simulink model "Control_model_10DOF_fin"  (R2016b)
settings: Solver=FixedStepAuto  StartTime=0.0  StopTime=10  FixedStep=0.0001  RelTol=1e-3
InitFcn:
  | Initialisation_ctr_10DOF_fin
values from neighbouring files (symbols this model uses):
  COM_Parameters = [-lpelvis/2;r2;0]    [Initialisation_ctr_10DOF_fin.m]
  DH_Parameters = [hfoot 0 ... (first row only)    [Initialisation_ctr_10DOF_fin.m]
  dTrunk = trunklbd(3)    [Initialisation_ctr_10DOF_fin.m]
  dxFootSM = dxFoot    [Initialisation_ctr_10DOF_fin.m]
  dxTrunk = 0.1    [Initialisation_ctr_10DOF_fin.m]
  Foot_Parameters = [0;-(lFoot/2-lHeel);0]    [Initialisation_ctr_10DOF_fin.m]
  HAA2HEE = [0; 0; 0.001]    [Initialisation_ctr_10DOF_fin.m]
  HEE2HFE = 0.5*[0.2; 0; 0]    [Initialisation_ctr_10DOF_fin.m]
  height_vrp = CoM_position(1)    [Initialisation_ctr_10DOF_fin.m]
  hTrunk = trunklbd(1)    [Initialisation_ctr_10DOF_fin.m]
  initial_CoM_position = R*CoM_position    [Initialisation_ctr_10DOF_fin.m]
  initial_CoM_velocity = [0;0;0]    [Initialisation_ctr_10DOF_fin.m]
  initial_left_foot = [0;0;-stance_width/2]    [Initialisation_ctr_10DOF_fin.m]
  initial_right_foot = [0;0;stance_width/2]    [Initialisation_ctr_10DOF_fin.m]
  initial_RorL = 0    [Initialisation_ctr_10DOF_fin.m]
  jointsinitial = [9;-15;6;0;0;6;-15;9]/180*pi    [Initialisation_ctr_10DOF_fin.m]
  K_DCM = 4.3*[1 0 0 ... (first row only)    [Initialisation_ctr_10DOF_fin.m]
  kD_left = mbody*[0.95 0 0 0 ... (first row only)    [Initialisation_ctr_10DOF_fin.m]
  kD_right = mbody*[0.12 0 0 0 ... (first row only)    [Initialisation_ctr_10DOF_fin.m]
  kI_left = mbody*[35 0 0 0 ... (first row only)    [Initialisation_ctr_10DOF_fin.m]
  kI_right = mbody*[38.2 0 0 0 ... (first row only)    [Initialisation_ctr_10DOF_fin.m]
  kP_left = mbody*[75 0 0 0 ... (first row only)    [Initialisation_ctr_10DOF_fin.m]
  kP_right = mbody*[5.6 0 0 0 ... (first row only)    [Initialisation_ctr_10DOF_fin.m]
  Lenght = [lShank;lThigh]    [Initialisation_ctr_10DOF_fin.m]
  lFootSM = lFoot    [Initialisation_ctr_10DOF_fin.m]
  lpelvis = wPelvis    [Initialisation_ctr_10DOF_fin.m]
  mass = mbody    (= 60)    [Initialisation_ctr_10DOF_fin.m]
  Masses = [mThigh; mShank; mTrunk]    [Initialisation_ctr_10DOF_fin.m]
  nb_step = 4    [Initialisation_ctr_10DOF_fin.m]
  nb_step_pattern = 20    [Initialisation_ctr_10DOF_fin.m]
  Pelvis_Parameters = [-lpelvis/2;hTrunk/2;0]    [Initialisation_ctr_10DOF_fin.m]
  stance_width = lpelvis    [Initialisation_ctr_10DOF_fin.m]
  stride_lenght = 0.50    (= 0.5)    [Initialisation_ctr_10DOF_fin.m]
  T_DS = time_DS    (= 0.4)    [Initialisation_ctr_10DOF_fin.m]
  T_IT = time_DS    (= 0.4)    [Initialisation_ctr_10DOF_fin.m]
  T_SS = time_swing    (= 1.6)    [Initialisation_ctr_10DOF_fin.m]
  time_DS = (time_stance-time_swing)/2    (= 0.4)    [Initialisation_ctr_10DOF_fin.m]
  time_stance = 60/100*time_stride    (= 2.4)    [Initialisation_ctr_10DOF_fin.m]
  time_step = time_stride/2    (= 2)    [Initialisation_ctr_10DOF_fin.m]
  time_swing = 40/100*time_stride    (= 1.6)    [Initialisation_ctr_10DOF_fin.m]
  validity_angle = [-20*pi/180 20*pi/180 ... (first row only)    [Initialisation_ctr_10DOF_fin.m]
  wTrunk = trunklbd(2)    [Initialisation_ctr_10DOF_fin.m]
  x4CoM = CoM_position(1)-XR4(1)    [Initialisation_ctr_10DOF_fin.m]
undefined symbols (not defined in the file or in its folder): dsegment, hFoot, l, lFoot, omega0_x, omega0_z, rho, wPelvis, X, Xp_x, Xp_z, Y, Z
undefined symbols (not defined in the file): k_grf, lShankSM, lThighSM, mShank, mThigh
libraries: nesl_utility x247, sm_lib x215, dspindex x12, FootPlacementLibrary x8, dspsigops x4, dspswit3 x1
(part 14 of 18)

== matlab function Control_model_10DOF_fin/10DoF Walker SimMechanics Model/Knee FE/MATLAB Function ==
  data: joint input; velocity input; desired_torque input; torque output; validity_angle parameter
function torque = fcn(joint,velocity,desired_torque,validity_angle)

kp=900;
kv=0.008;

min=validity_angle(2,1);
max=validity_angle(2,2);

if joint<=min
    torque=kp*(min-joint)-kv*velocity;
    if torque<=0
        torque=desired_torque;
    end
elseif joint>=max
    torque=kp*(max-joint)-kv*velocity;
    if torque>=0
        torque=desired_torque;
    end
else
    torque=desired_torque;
end

== matlab function Control_model_10DOF_fin/10DoF Walker SimMechanics Model/Knee FE1/MATLAB Function ==
  data: joint input; velocity input; desired_torque input; torque output; validity_angle parameter
function torque = fcn(joint,velocity,desired_torque,validity_angle)

kp=900;
kv=0.008;

min=validity_angle(7,1);
max=validity_angle(7,2);

if joint<=min
    torque=kp*(min-joint)-kv*velocity;
    if torque<=0
        torque=desired_torque;
    end
elseif joint>=max
    torque=kp*(max-joint)-kv*velocity;
    if torque>=0
        torque=desired_torque;
    end
else
    torque=desired_torque;
end

== matlab function Control_model_10DOF_fin/Control/Double_Support/Left stance phase1/Subsystem/MATLAB Function1 ==
  data: r_vrp_W input size=3; TWR input; TWL input; lFoot parameter; dsegment parameter; new_vrp_W output; alpha output
function [new_vrp_W,alpha]  = support_polygon(r_vrp_W,TWR,TWL,lFoot,dsegment)


RWL=TWL(1:3,1:3);
Left_foot_position=TWL(1:3,4);
Right_foot_position=TWR(1:3,4);

p=85/100;

R1W=Right_foot_position+RWL*[0;-lFoot/2;-dsegment/2]*p;
R2W=Right_foot_position+RWL*[0;-lFoot/2;dsegment/2]*p;
R3W=Right_foot_position+RWL*[0;lFoot/2;dsegment/2]*p;
R4W=Right_foot_position+RWL*[0;lFoot/2;-dsegment/2]*p;

L1W=Left_foot_position+RWL*[0;-lFoot/2;-dsegment/2]*p;
L2W=Left_foot_position+RWL*[0;-lFoot/2;dsegment/2]*p;
L3W=Left_foot_position+RWL*[0;lFoot/2;dsegment/2]*p;
L4W=Left_foot_position+RWL*[0;lFoot/2;-dsegment/2]*p;

dR=norm(r_vrp_W-Right_foot_position);
dL=norm(r_vrp_W-Left_foot_position);

alpha=dR/(dR+dL);
% if Right_foot_position(2)>0
%     alpha=1;
% end

% Projection on the ground
R1W(2)=0;
R2W(2)=0;
R3W(2)=0;
R4W(2)=0;

L1W(2)=0;
L2W(2)=0;
L3W(2)=0;
L4W(2)=0;

% New frame

x=1/norm(L1W-L4W)*(L1W-L4W);
y=[0;1;0];
z=1/norm(L2W-L1W)*(L2W-L1W);

R=[x,y,z];

% Points on the Left foot origin and new frame


L1=R.'*(L1W-Left_foot_position);
L2=R.'*(L2W-Left_foot_position);
L3=R.'*(L3W-Left_foot_position);
L4=R.'*(L4W-Left_foot_position);

% VRP and DCM on the left foot origin and new frame

r_vrp=R.'*(r_vrp_W-Left_foot_position);


outside=1;

if r_vrp(1)<L1(1) && r_vrp(3)>L1(3) && r_vrp(1)>L3(1) && r_vrp(3)<L3(3)
    outside=0;
    alpha=0;
end

cas=0;

new_vrp=r_vrp;

if outside==1
    if r_vrp(1)>=L1(1) && r_vrp(3)<=L1(3)
        new_vrp(1)=L1(1);
        new_vrp(3)=L1(3);
    elseif r_vrp(1)>=L2(1) && r_vrp(3)>=L2(3)
        new_vrp(1)=L2(1);
        new_vrp(3)=L2(3);
    elseif r_vrp(1)>=L1(1)
        new_vrp(1)=L1(1);
    elseif r_vrp(1)<=L3(1) && r_vrp(3)>=L3(3)
        new_vrp(1)=L3(1);
        new_vrp(3)=L3(3);
    elseif r_vrp(3)>=L3(3)
        new_vrp(3)=L3(3);
    elseif r_vrp(1)<=L4(1) && r_vrp(3)<=L4(3)
        new_vrp(1)=L4(1);
        new_vrp(3)=L4(3);
    elseif r_vrp(1)<=L4(1)
        new_vrp(1)=L4(1);
    else
        new_vrp(3)=L4(3);
    end
end



new_vrp_W=R*new_vrp+Left_foot_position;

== matlab function Control_model_10DOF_fin/Control/Double_Support/Left stance phase1/Subsystem/MATLAB Function2 ==
  data: r_vrp input double size=[3 1]; Force_des output double size=[3 1]; r_CoM input double size=[3 1]; mass parameter double size=1; height_vrp parameter double size=1
function Force_des = Force_transformation(r_vrp,r_CoM, mass, height_vrp)
g=9.81;
Force_des = mass*g/height_vrp*(r_CoM-(r_vrp-[0;height_vrp;0]));

== matlab function Control_model_10DOF_fin/Control/Double_Support/Left stance phase1/Subsystem/MATLAB Function3 ==
  data: Force_des input double size=[3 1]; alpha input; Torques_des output; JcomR input; JcomL input; TWR input; TWL input; alpha output
function [Torques_des,alpha] = Force_to_Torques(Force_des,alpha,JcomR,JcomL,TWR,TWL)

XWR=TWR(1:3,4);
XWL=TWL(1:3,4);

RWR=TWR(1:3,1:3);
RWL=TWL(1:3,1:3);

% if XWR(2)>0
%     alpha=0;
% end

alpha=1;

Force_corrR=(alpha)*RWR.'*Force_des;

% JR=[JcomR(1,1) JcomR(1,3);
%     JcomR(2,1) JcomR(2,3);
%     JcomR(3,1) JcomR(3,3)];
JR=[JcomR(1,1) JcomR(1,3);
    JcomR(2,1) JcomR(2,3)];
% JR=[JcomR(1,3);
%     JcomR(2,3);
%     JcomR(3,3)];

Torques_right=JR.'*Force_corrR(1:2);


Force_corrL=(1-alpha)*RWL.'*Force_des;

% JL=[JcomL(1,6) JcomL(1,8);
%     JcomL(2,6) JcomL(2,8);
%     JcomL(3,6) JcomL(3,8)];
% JL=[JcomL(1,6);
%     JcomL(2,6);
%     JcomL(3,6)];

JL=[JcomL(1,6) JcomL(1,8);
    JcomL(2,6) JcomL(2,8)];

Torques_left=JL.'*Force_corrL(1:2);

Torques_des=[Torques_right;Torques_left];

end

== matlab function Control_model_10DOF_fin/Control/Double_Support/Left stance phase1/Subsystem/MATLAB Function4 ==
  data: r_vrp input double size=[3 1]; Force_des output double size=[3 1]; r_CoM input double size=[3 1]; TWR input; mass parameter double size=1; height_vrp parameter double size=1
function Force_des = Force_transformation(r_vrp,r_CoM,TWR, mass, height_vrp)
g=9.81;
Force_des = mass*g/height_vrp*(r_CoM-(r_vrp-[0;height_vrp;0]));

RWR=TWR(1:3,1:3);

Force_des_R=RWR.'*Force_des;
Force_des_R(1)=0;
Force_des_R(2)=0;

Force_des=RWR*Force_des_R;

== matlab function Control_model_10DOF_fin/Control/Double_Support/Left stance phase1/Subsystem/MATLAB Function5 ==
  data: r_vrp_W input size=3; TWR input; lFoot parameter; dsegment parameter; new_vrp_W output; outside output; cas output
function [new_vrp_W,outside,cas]  = support_polygon(r_vrp_W,TWR,lFoot,dsegment)

RWR=TWR(1:3,1:3);

Right_foot_position=TWR(1:3,4);

p=85/100;

R1W=Right_foot_position+RWR*[0;lFoot/2;dsegment/2]*p;
R2W=Right_foot_position+RWR*[0;lFoot/2;-dsegment/2]*p;
R3W=Right_foot_position+RWR*[0;-lFoot/2;-dsegment/2]*p;
R4W=Right_foot_position+RWR*[0;-lFoot/2;dsegment/2]*p;

% Projection on the ground
R1W(2)=0;
R2W(2)=0;
R3W(2)=0;
R4W(2)=0;

% New frame

x=1/norm(R1W-R4W)*(R1W-R4W);
y=[0;1;0];
z=1/norm(R2W-R1W)*(R2W-R1W);

R=[x,y,z];

% Points on the Right foot origin and new frame

R1=R.'*(R1W-Right_foot_position);
R2=R.'*(R2W-Right_foot_position);
R3=R.'*(R3W-Right_foot_position);
R4=R.'*(R4W-Right_foot_position);

% VRP and DCM on the left foot origin and new frame

r_vrp=R.'*(r_vrp_W-Right_foot_position);

outside=1;

if r_vrp(3)>R1(3) && r_vrp(1)<R1(1) && r_vrp(3)<R3(3) && r_vrp(1)>R3(1)
    outside=0;
end



cas=0;

new_vrp=r_vrp;

if outside==1
    if r_vrp(1)>=R1(1) && r_vrp(3)<=R1(3)
        new_vrp(1)=R1(1);
        new_vrp(3)=R1(3);
    elseif r_vrp(1)>=R2(1) && r_vrp(3)>=R2(3)
        new_vrp(1)=R2(1);
        new_vrp(3)=R2(3);
    elseif r_vrp(1)>=R1(1)
        new_vrp(1)=R1(1);
    elseif r_vrp(1)<=R3(1) && r_vrp(3)>=R3(3)
        new_vrp(1)=R3(1);
        new_vrp(3)=R3(3);
    elseif r_vrp(3)>=R3(3)
        new_vrp(3)=R3(3);
    elseif r_vrp(1)<=R4(1) && r_vrp(3)<=R4(3)
        new_vrp(1)=R4(1);
        new_vrp(3)=R4(3);
    elseif r_vrp(1)<=R4(1)
        new_vrp(1)=R4(1);
    else
        new_vrp(3)=R4(3);
    end
end

new_vrp_W=R*new_vrp+Right_foot_position;

== matlab function Control_model_10DOF_fin/Control/Double_Support/Left stance phase1/Subsystem/VRP based DCM tracking control ==
  data: r_extrapolated_CoM input double size=[3 1]; r_vrp output double size=[3 1]; DCM_velocity input double size=[3 1]; height_vrp parameter double size=1; DCM_position input double size=[3 1]; K_DCM parameter double size=[3 3]
function r_vrp = vrp_calcul(r_extrapolated_CoM,DCM_velocity,height_vrp, DCM_position, K_DCM)
%Gravity
g=9.81;
% K_DCM=0.5*[1 0 0;
% 0 1 0;
% 0 0 1];

r_vrp=r_extrapolated_CoM+K_DCM*sqrt(height_vrp/g)*(r_extrapolated_CoM-DCM_position)-sqrt(height_vrp/g)*DCM_velocity;

== matlab function Control_model_10DOF_fin/Control/Double_Support/Left stance phase1/Subsystem/extrapolated CoM calcul ==
  data: CoM_position input double size=[3 1]; r_extrapolate_CoM output double size=[3 1]; CoM_velocity input double size=[3 1]; height_vrp parameter double size=1
function r_extrapolate_CoM = DCM_calcul(CoM_position,CoM_velocity,height_vrp)
%Gravity
g=9.81;
r_extrapolate_CoM=CoM_position+sqrt(height_vrp/g)*CoM_velocity;

== matlab function Control_model_10DOF_fin/Control/Double_Support/Right stance phase/Subsystem/MATLAB Function ==
  data: r_vrp input double size=[3 1]; Force_des output double size=[3 1]; r_CoM input double size=[3 1]; mass parameter double size=1; height_vrp parameter double size=1
function Force_des = Force_transformation(r_vrp,r_CoM, mass, height_vrp)
g=9.81;
Force_des = mass*g/height_vrp*(r_CoM-(r_vrp-[0;height_vrp;0]));

== matlab function Control_model_10DOF_fin/Control/Double_Support/Right stance phase/Subsystem/MATLAB Function1 ==
  data: r_vrp_W input size=3; TWL input; lFoot parameter; dsegment parameter; new_vrp_W output; outside output; cas output
function [new_vrp_W,outside,cas]  = support_polygon(r_vrp_W,TWL,lFoot,dsegment)

RWL=TWL(1:3,1:3);
Left_foot_position=TWL(1:3,4);

p=85/100;

L1W=Left_foot_position+RWL*[0;-lFoot/2;-dsegment/2]*p;
L2W=Left_foot_position+RWL*[0;-lFoot/2;dsegment/2]*p;
L3W=Left_foot_position+RWL*[0;lFoot/2;dsegment/2]*p;
L4W=Left_foot_position+RWL*[0;lFoot/2;-dsegment/2]*p;

% Projection on the ground

L1W(2)=0;
L2W(2)=0;
L3W(2)=0;
L4W(2)=0;

% New frame

x=1/norm(L1W-L4W)*(L1W-L4W);
y=[0;1;0];
z=1/norm(L2W-L1W)*(L2W-L1W);

R=[x,y,z];

% Points on the Left foot origin and new frame

L1=R.'*(L1W-Left_foot_position);
L2=R.'*(L2W-Left_foot_position);
L3=R.'*(L3W-Left_foot_position);
L4=R.'*(L4W-Left_foot_position);

% VRP and DCM on the left foot origin and new frame

r_vrp=R.'*(r_vrp_W-Left_foot_position);


outside=1;

if r_vrp(1)<L1(1) && r_vrp(3)>L1(3) && r_vrp(1)>L3(1) && r_vrp(3)<L3(3)
    outside=0;
end

cas=0;

new_vrp=r_vrp;

if outside==1
    if r_vrp(1)>=L1(1) && r_vrp(3)<=L1(3)
        new_vrp(1)=L1(1);
        new_vrp(3)=L1(3);
    elseif r_vrp(1)>=L2(1) && r_vrp(3)>=L2(3)
        new_vrp(1)=L2(1);
        new_vrp(3)=L2(3);
    elseif r_vrp(1)>=L1(1)
        new_vrp(1)=L1(1);
    elseif r_vrp(1)<=L3(1) && r_vrp(3)>=L3(3)
        new_vrp(1)=L3(1);
        new_vrp(3)=L3(3);
    elseif r_vrp(3)>=L3(3)
        new_vrp(3)=L3(3);
    elseif r_vrp(1)<=L4(1) && r_vrp(3)<=L4(3)
        new_vrp(1)=L4(1);
        new_vrp(3)=L4(3);
    elseif r_vrp(1)<=L4(1)
        new_vrp(1)=L4(1);
    else
        new_vrp(3)=L4(3);
    end
end

new_vrp_W=R*new_vrp+Left_foot_position;

== matlab function Control_model_10DOF_fin/Control/Double_Support/Right stance phase/Subsystem/MATLAB Function2 ==
  data: r_vrp input double size=[3 1]; Force_des output double size=[3 1]; r_CoM input double size=[3 1]; TWL input; mass parameter double size=1; height_vrp parameter double size=1
function Force_des = Force_transformation(r_vrp,r_CoM,TWL, mass, height_vrp)
g=9.81;
Force_des = mass*g/height_vrp*(r_CoM-(r_vrp-[0;height_vrp;0]));
RWL=TWL(1:3,1:3);

Force_des_L=RWL.'*Force_des;
Force_des_L(1)=0;
Force_des_L(2)=0;

Force_des =RWL*Force_des_L;

== matlab function Control_model_10DOF_fin/Control/Double_Support/Right stance phase/Subsystem/MATLAB Function3 ==
  data: Force_des input double size=[3 1]; alpha input; Torques_des output; JcomR input; JcomL input; TWR input; TWL input; alpha output
function [Torques_des,alpha] = Force_to_Torques(Force_des,alpha,JcomR,JcomL,TWR,TWL)

XWR=TWR(1:3,4);
XWL=TWL(1:3,4);

RWR=TWR(1:3,1:3);
RWL=TWL(1:3,1:3);

% if XWR(2)>0
%     alpha=0;
% end

Force_corrR=(alpha)*RWR.'*Force_des;
% 
% JR=[JcomR(1,1) JcomR(1,3);
%     JcomR(2,1) JcomR(2,3);
%     JcomR(3,1) JcomR(3,3)];

JR=[JcomR(1,1) JcomR(1,3);
    JcomR(2,1) JcomR(2,3)];

% JR=[JcomR(1,3);
%     JcomR(2,3);
%     JcomR(3,3)];

Torques_right=JR.'*Force_corrR(1:2);


Force_corrL=(1-alpha)*RWL.'*Force_des;

% JL=[JcomL(1,6) JcomL(1,8);
%     JcomL(2,6) JcomL(2,8);
%     JcomL(3,6) JcomL(3,8)];
JL=[JcomL(1,6) JcomL(1,8);
    JcomL(2,6) JcomL(2,8)];
% JL=[JcomL(1,6);
%     JcomL(2,6);
%     JcomL(3,6)];

Torques_left=JL.'*Force_corrL(1:2);

Torques_des=[Torques_right;Torques_left];

end

== matlab function Control_model_10DOF_fin/Control/Double_Support/Right stance phase/Subsystem/MATLAB Function5 ==
  data: r_vrp_W input size=3; TWR input; TWL input; lFoot parameter; dsegment parameter; new_vrp_W output; alpha output; cas output
function [new_vrp_W,alpha,cas]  = support_polygon(r_vrp_W,TWR,TWL,lFoot,dsegment)

RWR=TWR(1:3,1:3);
Right_foot_position=TWR(1:3,4);
Left_foot_position=TWL(1:3,4);

R1W=Right_foot_position+RWR*[0;lFoot/2;dsegment/2];
R2W=Right_foot_position+RWR*[0;lFoot/2;-dsegment/2];
R3W=Right_foot_position+RWR*[0;-lFoot/2;-dsegment/2];
R4W=Right_foot_position+RWR*[0;-lFoot/2;dsegment/2];

dR=norm(r_vrp_W-Right_foot_position);
dL=norm(r_vrp_W-Left_foot_position);

alpha=dR/(dR+dL);

% Projection on the ground
R1W(2)=0;
R2W(2)=0;
R3W(2)=0;
R4W(2)=0;

% New frame

x=1/norm(R1W-R4W)*(R1W-R4W);
y=[0;1;0];
z=1/norm(R2W-R1W)*(R2W-R1W);

R=[x,y,z];

% Points on the Right foot origin and new frame

R1=R.'*(R1W-Right_foot_position);
R2=R.'*(R2W-Right_foot_position);
R3=R.'*(R3W-Right_foot_position);
R4=R.'*(R4W-Right_foot_position);

% VRP and DCM on the left foot origin and new frame

r_vrp=R.'*(r_vrp_W-Right_foot_position);

outside=1;

if r_vrp(3)>R1(3) && r_vrp(1)<R1(1) && r_vrp(3)<R3(3) && r_vrp(1)>R3(1)
    outside=0;
    alpha=0;
% elseif r_vrp(3)>L1(3) && r_vrp(1)<L1(1) && r_vrp(3)<L3(3) && r_vrp(1)>L3(1)
%     outside=0;
%     alpha=1;
end

cas=0;

new_vrp=r_vrp;

if outside==1
    if r_vrp(1)>=R1(1) && r_vrp(3)<=R1(3)
        new_vrp(1)=R1(1);
        new_vrp(3)=R1(3);
    elseif r_vrp(1)>=R2(1) && r_vrp(3)>=R2(3)
        new_vrp(1)=R2(1);
        new_vrp(3)=R2(3);
    elseif r_vrp(1)>=R1(1)
        new_vrp(1)=R1(1);
    elseif r_vrp(1)<=R3(1) && r_vrp(3)>=R3(3)
        new_vrp(1)=R3(1);
        new_vrp(3)=R3(3);
    elseif r_vrp(3)>=R3(3)
        new_vrp(3)=R3(3);
    elseif r_vrp(1)<=R4(1) && r_vrp(3)<=R4(3)
        new_vrp(1)=R4(1);
        new_vrp(3)=R4(3);
    elseif r_vrp(1)<=R4(1)
        new_vrp(1)=R4(1);
    else
        new_vrp(3)=R4(3);
    end
end

new_vrp_W=R*new_vrp+Right_foot_position;

== matlab function Control_model_10DOF_fin/Control/Double_Support/Right stance phase/Subsystem/VRP based DCM tracking control ==
  data: r_extrapolated_CoM input double size=[3 1]; r_vrp output double size=[3 1]; DCM_velocity input double size=[3 1]; height_vrp parameter double size=1; DCM_position input double size=[3 1]; K_DCM parameter double size=[3 3]
function r_vrp = vrp_calcul(r_extrapolated_CoM,DCM_velocity,height_vrp, DCM_position, K_DCM)
%Gravity
g=9.81;

% K_DCM=2*[1 0 0;
%     0 1 0;
%     0 0 1];

r_vrp=r_extrapolated_CoM+K_DCM*sqrt(height_vrp/g)*(r_extrapolated_CoM-DCM_position)-sqrt(height_vrp/g)*DCM_velocity;

== matlab function Control_model_10DOF_fin/Control/Double_Support/Right stance phase/Subsystem/extrapolated CoM calcul ==
  data: CoM_position input double size=[3 1]; r_extrapolate_CoM output double size=[3 1]; CoM_velocity input double size=[3 1]; height_vrp parameter double size=1
function r_extrapolate_CoM = DCM_calcul(CoM_position,CoM_velocity,height_vrp)
%Gravity
g=9.81;
r_extrapolate_CoM=CoM_position+sqrt(height_vrp/g)*CoM_velocity;

== matlab function Control_model_10DOF_fin/Control/Finish_Swing_Phase/Left Swing // Right Stance/Left Swing leg control/Left ==
  data: desired_joint_angle output size=4; TR5 input; TR8 input; TR9 input; TRL input; TWR input; swing_state input; desired_knee_angle input; DH_Parameters parameter; actual_joint_angle input size=4; ok output; cas output; Foot_Parameters parameter
function [desired_joint_angle,ok,cas] = Backward_Kinematics_swing(TR5,TR8,TR9,TRL,TWR,swing_state,desired_knee_angle,DH_Parameters,actual_joint_angle,Foot_Parameters)


RWR=TWR(1:3,1:3);
XWR=TWR(1:3,4);

XWfoot=swing_state(1:3);

XRfoot=RWR.'*(XWfoot-XWR);

yfoot=XRfoot(2)+Foot_Parameters(2);
zfoot=XRfoot(3);
% desired_knee_angle=swing_state(4);

actual_theta7=actual_joint_angle(3);
theta7=desired_knee_angle;

a0=DH_Parameters(1,1);
d0=DH_Parameters(1,2);
a1=DH_Parameters(2,1);
d1=DH_Parameters(2,2);
a2=DH_Parameters(3,1);
d2=DH_Parameters(3,2);
a3=DH_Parameters(4,1);
d3=DH_Parameters(4,2);
a4=DH_Parameters(5,1);
d4=DH_Parameters(5,2);
a5=DH_Parameters(6,1);
d5=DH_Parameters(6,2);
a6=DH_Parameters(7,1);
d6=DH_Parameters(7,2);
a7=DH_Parameters(8,1);
d7=DH_Parameters(8,2);
a8=DH_Parameters(9,1);
d8=DH_Parameters(9,2);


% zhip=TR5(3,4);
yhip=TR5(2,4);
xhip=TR5(1,4);


%%%%%%%%%%%%%%% theta6 %%%%%%%%%%%%%%%

angle1= 2*atan((a6 + (a7^2 + a6^2 + 2*a6*a7*cos(actual_theta7))^(1/2) + a7*cos(actual_theta7))/(a7*sin(actual_theta7)));
 
if yhip>=0 && yhip<=yfoot
    ok=1;
    angle2=atan((abs(yfoot)-abs(yhip))/abs(xhip))+atan(abs(yhip)/abs(xhip));
    theta6=angle1+angle2;
elseif yhip<=0 && 0<=yfoot
    ok=2;
    angle2=atan((abs(yfoot)+abs(yhip))/abs(xhip))-atan(abs(yhip)/abs(xhip));
    theta6=angle1+angle2;
elseif yfoot<=yhip && yhip<=0
    ok=3;
    angle2=atan((abs(yfoot)-abs(yhip))/abs(xhip))+atan(abs(yhip)/abs(xhip));
    theta6=angle1-angle2;
elseif yfoot<=0 && 0<=yhip
    ok=4;
    angle2=atan((abs(yfoot)+abs(yhip))/abs(xhip))-atan(abs(yhip)/abs(xhip));
    theta6=angle1-angle2;
elseif 0<=yfoot && yfoot<=yhip
    ok=5;
    angle2=atan(abs(yhip)/abs(xhip))-atan((abs(yhip)-abs(yfoot))/abs(xhip));
    theta6=angle1+angle2;
else
    ok=6;
    angle2=atan(abs(yhip)/abs(xhip))-atan((abs(yhip)-abs(yfoot))/abs(xhip));
    theta6=angle1-angle2;
end


%%%%%%%%%%%%%%% theta4 %%%%%%%%%%%%%%%

xR5=TR5(1,4);
% yR5=TR5(2,4);
zR5=TR5(3,4);

xR8=TR8(1,4);
% yR8=TR8(2,4);
zR8=TR8(3,4);

actual_theta5=actual_joint_angle(1);

cas=0;

if zR5<=zfoot && zR8<=zfoot
    cas=1;
    alpha8=atan((zR5-zR8)/(xR5-xR8));
    alphaFoot=atan((zR5-zfoot)/xR5);
    error=alpha8+alphaFoot;
    theta5=actual_theta5-error;
%     if error <=0
%         theta5=actual_theta5-error;
%     else
%         theta5=actual_theta5+error;
%     end
elseif zR5>=zfoot && zR8>=zfoot && zR8<zR5
    cas=2;
    alpha8=atan((zR5-zR8)/(xR5-xR8));
    alphaFoot=atan((zR5-zfoot)/xR5);
    error=alphaFoot-alpha8;
    theta5=actual_theta5-error;
elseif zR5>=zfoot && zR8>zR5
    cas=3;
    alpha8=atan((zR8-zR5)/(xR5-xR8));
    alphaFoot=atan((zR5-zfoot)/xR5);
    error=alphaFoot+alpha8;
    theta5=actual_theta5-error;
elseif zR5<=zfoot && zR8<zR5
    cas=4;
    alpha8=atan((zR5-zR8)/(xR5-xR8));
    alphaFoot=atan((zfoot-zR5)/xR5);
    error=alphaFoot+alpha8;
    theta5=actual_theta5+error;
elseif zR5<=zfoot && zR8>=zR5 && zR8<=zfoot
    cas=5;
    alpha8=atan((zR8-zR5)/(xR5-xR8));
    alphaFoot=atan((zfoot-zR5)/xR5);
    error=alphaFoot-alpha8;
    theta5=actual_theta5+error;
else
    cas=6;
    alpha8=atan((zR8-zR5)/(xR5-xR8));
    alphaFoot=atan((zfoot-zR5)/xR5);
    error=-alphaFoot+alpha8;
    theta5=actual_theta5-error;
%     if error>=0
%         theta5=actual_theta5-error;
%     else
%         theta5=actual_theta5+error;
%     end
end

%%%%%%%%%%%%%%%% theta8 %%%%%%%%%%%%%%%%%%%%

actual_theta8=actual_joint_angle(4);

xR9=TR9(1,4);
yR9=TR9(2,4);

xRL=TRL(1,4);
yRL=TRL(2,4);

error=atan((xRL-xR9)/(yRL-yR9));
theta8=actual_theta8-error;

desired_joint_angle=[theta5;theta6;theta7;theta8];

== matlab function Control_model_10DOF_fin/Control/Finish_Swing_Phase/Left Swing // Right Stance/MATLAB Function ==
  data: swing_state input; new_swing_state output; foot_adjust input
function new_swing_state = fcn(swing_state,foot_adjust)

zfoot=swing_state(3);
new_swing_state=swing_state;
if foot_adjust(3)<zfoot
    new_swing_state(3)=foot_adjust(3);
end

== matlab function Control_model_10DOF_fin/Control/Finish_Swing_Phase/Left Swing // Right Stance/Right Stance leg control/DCM calcul ==
  data: CoM_position input double size=[3 1]; r_extrapolated_CoM output double size=[3 1]; CoM_velocity input double size=[3 1]; height_vrp parameter double size=1
function r_extrapolated_CoM = DCM_calcul(CoM_position,CoM_velocity,height_vrp)
%Gravity
g=9.81;
r_extrapolated_CoM=CoM_position+sqrt(height_vrp/g)*CoM_velocity;

== matlab function Control_model_10DOF_fin/Control/Finish_Swing_Phase/Left Swing // Right Stance/Right Stance leg control/MATLAB Function ==
  data: r_vrp input double size=[3 1]; Force_des output double size=[3 1]; r_CoM input double size=[3 1]; mass parameter double size=1; height_vrp parameter double size=1
function Force_des = Force_transformation(r_vrp,r_CoM, mass, height_vrp)
g=9.81;
Force_des = mass*g/height_vrp*(r_CoM-(r_vrp-[0;height_vrp;0]));

== matlab function Control_model_10DOF_fin/Control/Finish_Swing_Phase/Left Swing // Right Stance/Right Stance leg control/MATLAB Function1 ==
  data: Force_des_W input double size=[3 1]; JcomR input; Torques_des output double; TWR input
function Torques_des   = Force_to_Torques(Force_des_W,JcomR,TWR)

RWR=TWR(1:3,1:3);

Force_des_R=RWR.'*Force_des_W;
% Force_des_R(3)=0;

% J=[JcomR(1,1),JcomR(1,3),JcomR(1,4);
%     JcomR(2,1),JcomR(2,3),JcomR(2,4);
%     JcomR(3,1),JcomR(3,3),JcomR(3,4)];
% J=[JcomR(1,1),JcomR(1,3);
%     JcomR(2,1),JcomR(2,3);
%     JcomR(3,1),JcomR(3,3)];

J=[JcomR(1,1),JcomR(1,3);
    JcomR(2,1),JcomR(2,3)];

Torques_des=J.'*Force_des_R(1:2);

end

== matlab function Control_model_10DOF_fin/Control/Finish_Swing_Phase/Left Swing // Right Stance/Right Stance leg control/MATLAB Function2 ==
  data: r_vrp input double size=[3 1]; Force_des output double size=[3 1]; r_CoM input double size=[3 1]; TWR input; mass parameter double size=1; height_vrp parameter double size=1
function Force_des = Force_transformation(r_vrp,r_CoM,TWR, mass, height_vrp)
g=9.81;
Force_des = mass*g/height_vrp*(r_CoM-(r_vrp-[0;height_vrp;0]));

RWR=TWR(1:3,1:3);

Force_des_R=RWR.'*Force_des;
Force_des_R(1)=0;
Force_des_R(2)=0;

Force_des=RWR*Force_des_R;

== matlab function Control_model_10DOF_fin/Control/Finish_Swing_Phase/Left Swing // Right Stance/Right Stance leg control/MATLAB Function5 ==
  data: r_vrp_W input size=3; TWR input; lFoot parameter; dsegment parameter; new_vrp_W output; outside output; cas output
function [new_vrp_W,outside,cas]  = support_polygon(r_vrp_W,TWR,lFoot,dsegment)

RWR=TWR(1:3,1:3);

Right_foot_position=TWR(1:3,4);

p=85/100;

R1W=Right_foot_position+RWR*[0;lFoot/2;dsegment/2]*p;
R2W=Right_foot_position+RWR*[0;lFoot/2;-dsegment/2]*p;
R3W=Right_foot_position+RWR*[0;-lFoot/2;-dsegment/2]*p;
R4W=Right_foot_position+RWR*[0;-lFoot/2;dsegment/2]*p;

% Projection on the ground
R1W(2)=0;
R2W(2)=0;
R3W(2)=0;
R4W(2)=0;

% New frame

x=1/norm(R1W-R4W)*(R1W-R4W);
y=[0;1;0];
z=1/norm(R2W-R1W)*(R2W-R1W);

R=[x,y,z];

% Points on the Right foot origin and new frame

R1=R.'*(R1W-Right_foot_position);
R2=R.'*(R2W-Right_foot_position);
R3=R.'*(R3W-Right_foot_position);
R4=R.'*(R4W-Right_foot_position);

% VRP and DCM on the left foot origin and new frame

r_vrp=R.'*(r_vrp_W-Right_foot_position);

outside=1;

if r_vrp(3)>R1(3) && r_vrp(1)<R1(1) && r_vrp(3)<R3(3) && r_vrp(1)>R3(1)
    outside=0;
end



cas=0;

new_vrp=r_vrp;

if outside==1
    if r_vrp(1)>=R1(1) && r_vrp(3)<=R1(3)
        new_vrp(1)=R1(1);
        new_vrp(3)=R1(3);
    elseif r_vrp(1)>=R2(1) && r_vrp(3)>=R2(3)
        new_vrp(1)=R2(1);
        new_vrp(3)=R2(3);
    elseif r_vrp(1)>=R1(1)
        new_vrp(1)=R1(1);
    elseif r_vrp(1)<=R3(1) && r_vrp(3)>=R3(3)
        new_vrp(1)=R3(1);
        new_vrp(3)=R3(3);
    elseif r_vrp(3)>=R3(3)
        new_vrp(3)=R3(3);
    elseif r_vrp(1)<=R4(1) && r_vrp(3)<=R4(3)
        new_vrp(1)=R4(1);
        new_vrp(3)=R4(3);
    elseif r_vrp(1)<=R4(1)
        new_vrp(1)=R4(1);
    else
        new_vrp(3)=R4(3);
    end
end

new_vrp_W=R*new_vrp+Right_foot_position;

== matlab function Control_model_10DOF_fin/Control/Finish_Swing_Phase/Left Swing // Right Stance/Right Stance leg control/VRP based DCM tracking control ==
  data: r_extrapolated_CoM input double size=[3 1]; r_vrp output double size=[3 1]; DCM_velocity input double size=[3 1]; height_vrp parameter double size=1; DCM_position input double size=[3 1]; K_DCM parameter double size=[3 3]
function r_vrp = vrp_calcul(r_extrapolated_CoM,DCM_velocity,height_vrp, DCM_position, K_DCM)
%Gravity
g=9.81;

% K_DCM=2*[1 0 0;
% 0 1 0;
% 0 0 1];

r_vrp=r_extrapolated_CoM+K_DCM*sqrt(height_vrp/g)*(r_extrapolated_CoM-DCM_position)-sqrt(height_vrp/g)*DCM_velocity;

== matlab function Control_model_10DOF_fin/Control/Finish_Swing_Phase/Right Swing // Left Stance1/MATLAB Function ==
  data: swing_state input; new_swing_state output; foot_adjust input
function new_swing_state = fcn(swing_state,foot_adjust)

zfoot=swing_state(3);
new_swing_state=swing_state;
if foot_adjust(3)>zfoot
    new_swing_state(3)=foot_adjust(3);
end

== matlab function Control_model_10DOF_fin/Control/Finish_Swing_Phase/Right Swing // Left Stance1/Right Swing leg control/Right ==
  data: desired_joint_angle output size=4; TL4 input; TL1 input; TL0 input; TLR input; TWL input; swing_state input; desired_knee_angle input; DH_Parameters parameter; actual_joint_angle input size=4; ok output; cas output; Foot_Parameters parameter
function [desired_joint_angle,ok,cas] = Backward_Kinematics_swing(TL4,TL1,TL0,TLR,TWL,swing_state,desired_knee_angle,DH_Parameters,actual_joint_angle,Foot_Parameters)


RWL=TWL(1:3,1:3);
XWL=TWL(1:3,4);

XWfoot=swing_state(1:3);

XLfoot=RWL.'*(XWfoot-XWL);

yfoot=XLfoot(2)-Foot_Parameters(2);
zfoot=XLfoot(3);
% desired_knee_angle=swing_state(4);

actual_theta2=actual_joint_angle(2);
theta2=desired_knee_angle;

a0=DH_Parameters(1,1);
d0=DH_Parameters(1,2);
a1=DH_Parameters(2,1);
d1=DH_Parameters(2,2);
a2=DH_Parameters(3,1);
d2=DH_Parameters(3,2);
a3=DH_Parameters(4,1);
d3=DH_Parameters(4,2);
a4=DH_Parameters(5,1);
d4=DH_Parameters(5,2);
a5=DH_Parameters(6,1);
d5=DH_Parameters(6,2);
a6=DH_Parameters(7,1);
d6=DH_Parameters(7,2);
a7=DH_Parameters(8,1);
d7=DH_Parameters(8,2);
a8=DH_Parameters(9,1);
d8=DH_Parameters(9,2);


% zhip=TL4(3,4);
yhip=TL4(2,4);
xhip=TL4(1,4);


%%%%%%%%%%%%%%% theta3 %%%%%%%%%%%%%%%

angle1= 2*atan((a2 - (a1^2 + a2^2 + 2*a1*a2*cos(actual_theta2))^(1/2) + a1*cos(actual_theta2))/(a1*sin(actual_theta2)));

if yhip<=0 && yhip>=yfoot
    ok=1;
    angle2=atan((abs(yfoot)-abs(yhip))/abs(xhip))+atan(abs(yhip)/abs(xhip));
    theta3=angle1+angle2;
elseif yhip>=0 && 0>=yfoot
    ok=2;
    angle2=atan((abs(yfoot)+abs(yhip))/abs(xhip))-atan(abs(yhip)/abs(xhip));
    theta3=angle1+angle2;
elseif yfoot>=yhip && yhip>=0
    ok=3;
    angle2=atan((abs(yfoot)-abs(yhip))/abs(xhip))+atan(abs(yhip)/abs(xhip));
    theta3=angle1-angle2;
elseif yfoot>=0 && 0>=yhip
    ok=4;
    angle2=atan((abs(yfoot)+abs(yhip))/abs(xhip))-atan(abs(yhip)/abs(xhip));
    theta3=angle1+angle2;
elseif 0>=yfoot && yfoot>=yhip
    ok=5;
    angle2=atan(abs(yhip)/abs(xhip))-atan((abs(yhip)-abs(yfoot))/abs(xhip));
    theta3=angle1-angle2;
else
    ok=6;
    angle2=atan(abs(yhip)/abs(xhip))-atan((abs(yhip)-abs(yfoot))/abs(xhip));
    theta3=angle1+angle2;
end


%%%%%%%%%%%%%%% theta4 %%%%%%%%%%%%%%%

% xhip=TL4(1,4);
% % yL4=TL4(2,4);
% zhip=-TL4(3,4);
% 
% xankle=TL1(1,4);
% % yL1=TL1(2,4);
% zankle=-TL1(3,4);
% 
% xfoot=0;
% 
% actual_theta4=actual_joint_angle(4);
% 
% cas=0;
% 
% if zankle<=zfoot && zfoot<=zhip
%     cas=1
%     error=atan((zhip-zankle)/(xhip-xankle))-atan((zhip-zfoot)/(xhip-xfoot));
%     theta4=actual_theta4+error;
% elseif zfoot<=zankle && zankle<=zhip
%     cas=2;
%     error=atan((zhip-zfoot)/(xhip-xfoot))-atan((zhip-zankle)/(xhip-xankle));
%     theta4=actual_theta4-error;
% elseif zfoot<=zhip && zhip<=zankle
%     cas=3;
%     error=atan((zankle-zhip)/(xhip-xankle))+atan((zhip-zankle)/(xhip-xankle));
%     theta4=actual_theta4-error;
% elseif zhip<=zfoot && zfoot<=zankle
%     cas=4;
%     error=atan((zankle-zhip)/(xhip-xankle))-atan((zfoot-zhip)/(xfoot-xhip));
%     theta4=actual_theta4-error;
% elseif zankle<=zhip && zhip<=zfoot
%     cas=5;
%     error=atan((zhip-zankle)/(xhip-xankle))+atan((zfoot-zhip)/(xhip-xfoot));
%     theta4=actual_theta4+error;
% else
%     cas=6;
%     error=atan((zfoot-zhip)/(xhip-xfoot))-atan((zankle-zhip)/(xhip-xankle));
%     theta4=actual_theta4+error;
% end
% 
% theta4=actual_theta4;

xL4=TL4(1,4);
% yL4=TL4(2,4);
zL4=TL4(3,4);

xL0=TL1(1,4);
% yL1=TL1(2,4);
zL1=TL1(3,4);

actual_theta4=actual_joint_angle(4);

cas=0;

if zL4<=zfoot && zL1<=zfoot
    cas=1;
    alpha1=atan((zL4-zL1)/(xL4-xL0));
    alphaFoot=atan((zL4-zfoot)/xL4);
    error=alpha1+alphaFoot;
    theta4=actual_theta4+error;
%     if error <=0
%         theta5=actual_theta5-error;
%     else
%         theta5=actual_theta5+error;
%     end
elseif zL4>=zfoot && zL1>=zfoot && zL1<zL4
    cas=2;
    alpha1=atan((zL4-zL1)/(xL4-xL0));
    alphaFoot=atan((zL4-zfoot)/xL4);
    error=alphaFoot-alpha1;
    theta4=actual_theta4+error;
elseif zL4>=zfoot && zL1>zL4
    cas=3;
    alpha1=atan((zL1-zL4)/(xL4-xL0));
    alphaFoot=atan((zL4-zfoot)/xL4);
    error=alphaFoot+alpha1;
    theta4=actual_theta4+error;
elseif zL4<=zfoot && zL1<zL4
    cas=4;
    alpha1=atan((zL4-zL1)/(xL4-xL0));
    alphaFoot=atan((zfoot-zL4)/xL4);
    error=alphaFoot+alpha1;
    theta4=actual_theta4-error;
elseif zL4<=zfoot && zL1>=zL4 && zL1<=zfoot
    cas=5;
    alpha1=atan((zL1-zL4)/(xL4-xL0));
    alphaFoot=atan((zfoot-zL4)/xL4);
    error=alphaFoot-alpha1;
    theta4=actual_theta4-error;
else
    cas=6;
    alpha1=atan((zL1-zL4)/(xL4-xL0));
    alphaFoot=atan((zfoot-zL4)/xL4);
    error=-alphaFoot+alpha1;
    theta4=actual_theta4+error;
%     if error>=0
%         theta5=actual_theta5-error;
%     else
%         theta5=actual_theta5+error;
%     end
end



%%%%%%%%%%%%%%%% theta1 %%%%%%%%%%%%%%%%%%%%

% actual_theta1=actual_joint_angle(1);
% 
% xL0=TL0(1,4);
% yL0=TL0(2,4);
% 
% xLR=TLR(1,4);
% yLR=TLR(2,4);
% 
% X0R=TLR(1:3,4)-TL0(1:3,4);
% 
% xerror=abs(X0R(1));
% yerror=abs(X0R(2));
% 
% error_ankle=atan(xerror/yerror);
% theta1=actual_theta1+error_ankle;

actual_theta1=actual_joint_angle(1);

xL0=TL0(1,4);
yL0=TL0(2,4);

xLR=TLR(1,4);
yLR=TLR(2,4);

error=atan((xLR-xL0)/(yLR-yL0));
theta1=actual_theta1+error;


desired_joint_angle=[theta1;theta2;theta3;theta4];

== matlab function Control_model_10DOF_fin/Control/Finish_Swing_Phase/Right Swing // Left Stance1/Stance leg control/DCM calcul ==
  data: CoM_position input double size=[3 1]; r_DCM output double size=[3 1]; CoM_velocity input double size=[3 1]; height_vrp parameter double size=1
function r_DCM = DCM_calcul(CoM_position,CoM_velocity,height_vrp)
%Gravity
g=9.81;

r_DCM=CoM_position+sqrt(height_vrp/g)*CoM_velocity;

== matlab function Control_model_10DOF_fin/Control/Finish_Swing_Phase/Right Swing // Left Stance1/Stance leg control/MATLAB Function ==
  data: r_vrp input double size=[3 1]; Force_des output double size=[3 1]; r_CoM input double size=[3 1]; mass parameter double size=1; height_vrp parameter double size=1
function Force_des = Force_transformation(r_vrp,r_CoM, mass, height_vrp)
g=9.81;
Force_des = mass*g/height_vrp*(r_CoM-(r_vrp-[0;height_vrp;0]));

== matlab function Control_model_10DOF_fin/Control/Finish_Swing_Phase/Right Swing // Left Stance1/Stance leg control/MATLAB Function1 ==
  data: r_vrp input double size=[3 1]; Force_des output double size=[3 1]; r_CoM input double size=[3 1]; TWL input; mass parameter double size=1; height_vrp parameter double size=1
function Force_des = Force_transformation(r_vrp,r_CoM,TWL, mass, height_vrp)
g=9.81;
Force_des = mass*g/height_vrp*(r_CoM-(r_vrp-[0;height_vrp;0]));
RWL=TWL(1:3,1:3);

Force_des_L=RWL.'*Force_des;
Force_des_L(1)=0;
Force_des_L(2)=0;

Force_des =RWL*Force_des_L;

== matlab function Control_model_10DOF_fin/Control/Finish_Swing_Phase/Right Swing // Left Stance1/Stance leg control/MATLAB Function2 ==
  data: Force_des input double size=[3 1]; JcomL input; Torques_des output double; TWL input
function Torques_des   = Force_to_Torques(Force_des,JcomL,TWL)

RWL=TWL(1:3,1:3);

% J=[JcomL(1,5),JcomL(1,6),JcomL(1,8);
%     JcomL(2,5),JcomL(2,6),JcomL(2,8);
%     JcomL(3,5),JcomL(3,6),JcomL(3,8)];

% J=[JcomL(1,6),JcomL(1,8);
%     JcomL(2,6),JcomL(2,8);
%     JcomL(3,6),JcomL(3,8)];
J=[JcomL(1,6),JcomL(1,8);
    JcomL(2,6),JcomL(2,8)];

Force_des_L=RWL.'*Force_des;

Torques_des=J.'*Force_des_L(1:2);
% Torques_des(1)=-Torques_des(1);
% Torques_des(2)=-Torques_des(2);



end

== matlab function Control_model_10DOF_fin/Control/Finish_Swing_Phase/Right Swing // Left Stance1/Stance leg control/MATLAB Function5 ==
  data: r_vrp_W input size=3; TWL input; lFoot parameter; dsegment parameter; new_vrp_W output; outside output; cas output
function [new_vrp_W,outside,cas]  = support_polygon(r_vrp_W,TWL,lFoot,dsegment)

RWL=TWL(1:3,1:3);
Left_foot_position=TWL(1:3,4);

p=85/100;

L1W=Left_foot_position+RWL*[0;-lFoot/2;-dsegment/2]*p;
L2W=Left_foot_position+RWL*[0;-lFoot/2;dsegment/2]*p;
L3W=Left_foot_position+RWL*[0;lFoot/2;dsegment/2]*p;
L4W=Left_foot_position+RWL*[0;lFoot/2;-dsegment/2]*p;

% Projection on the ground

L1W(2)=0;
L2W(2)=0;
L3W(2)=0;
L4W(2)=0;

% New frame

x=1/norm(L1W-L4W)*(L1W-L4W);
y=[0;1;0];
z=1/norm(L2W-L1W)*(L2W-L1W);

R=[x,y,z];

% Points on the Left foot origin and new frame

L1=R.'*(L1W-Left_foot_position);
L2=R.'*(L2W-Left_foot_position);
L3=R.'*(L3W-Left_foot_position);
L4=R.'*(L4W-Left_foot_position);

% VRP and DCM on the left foot origin and new frame

r_vrp=R.'*(r_vrp_W-Left_foot_position);


outside=1;

if r_vrp(1)<L1(1) && r_vrp(3)>L1(3) && r_vrp(1)>L3(1) && r_vrp(3)<L3(3)
    outside=0;
end

cas=0;

new_vrp=r_vrp;

if outside==1
    if r_vrp(1)>=L1(1) && r_vrp(3)<=L1(3)
        new_vrp(1)=L1(1);
        new_vrp(3)=L1(3);
    elseif r_vrp(1)>=L2(1) && r_vrp(3)>=L2(3)
        new_vrp(1)=L2(1);
        new_vrp(3)=L2(3);
    elseif r_vrp(1)>=L1(1)
        new_vrp(1)=L1(1);
    elseif r_vrp(1)<=L3(1) && r_vrp(3)>=L3(3)
        new_vrp(1)=L3(1);
        new_vrp(3)=L3(3);
    elseif r_vrp(3)>=L3(3)
        new_vrp(3)=L3(3);
    elseif r_vrp(1)<=L4(1) && r_vrp(3)<=L4(3)
        new_vrp(1)=L4(1);
        new_vrp(3)=L4(3);
    elseif r_vrp(1)<=L4(1)
        new_vrp(1)=L4(1);
    else
        new_vrp(3)=L4(3);
    end
end

new_vrp_W=R*new_vrp+Left_foot_position;

== matlab function Control_model_10DOF_fin/Control/Finish_Swing_Phase/Right Swing // Left Stance1/Stance leg control/VRP based DCM tracking control ==
  data: r_DCM input double size=[3 1]; r_vrp output double size=[3 1]; DCM_velocity input double size=[3 1]; height_vrp parameter double size=1; DCM_position input double size=[3 1]; K_DCM parameter double size=[3 3]
function r_vrp = vrp_calcul(r_DCM,DCM_velocity,height_vrp, DCM_position, K_DCM)
%Gravity
g=9.81;

% K_DCM=2*[1 0 0;
% 0 1 0;
% 0 0 1];

r_vrp=r_DCM+K_DCM*sqrt(height_vrp/g)*(r_DCM-DCM_position)-sqrt(height_vrp/g)*DCM_velocity;

== matlab function Control_model_10DOF_fin/Control/Inititial_Transfert/Left stance phase1/Subsystem/MATLAB Function ==
  data: r_vrp input double size=[3 1]; Force_des output double size=[3 1]; r_CoM input double size=[3 1]; mass parameter double size=1; height_vrp parameter double size=1
function Force_des = Force_transformation(r_vrp,r_CoM, mass, height_vrp)
g=9.81;
Force_des = mass*g/height_vrp*(r_CoM-(r_vrp-[0;height_vrp;0]));

== matlab function Control_model_10DOF_fin/Control/Inititial_Transfert/Left stance phase1/Subsystem/MATLAB Function3 ==
  data: Force_des input double size=[3 1]; Torques_des output; JcomR input; JcomL input; TWR input; TWL input; alpha output; XRcom input; XLcom input
function [Torques_des,alpha] = Force_to_Torques(Force_des,JcomR,JcomL,TWR,TWL,XRcom,XLcom)

XWR=TWR(1:3,4);
XWL=TWL(1:3,4);

RWR=TWR(1:3,1:3);
RWL=TWL(1:3,1:3);


alpha=abs(XLcom(3))/(abs(XRcom(3))+abs(XLcom(3)));
% 
% dR=norm(XRcom);
% dL=norm(XLcom);
% 
% alpha=dL/(dR+dL);

Force_corrR=alpha*RWR.'*Force_des;

JR=[JcomR(1,1) JcomR(1,3);
    JcomR(2,1) JcomR(2,3);
    JcomR(3,1) JcomR(3,3)];

Torques_right=JR.'*Force_corrR;


Force_corrL=(1-alpha)*RWL.'*Force_des;

JL=[JcomL(1,6) JcomL(1,8);
    JcomL(2,6) JcomL(2,8);
    JcomL(3,6) JcomL(3,8)];

Torques_left=JL.'*Force_corrL;
% Torques_left(1)=-Torques_left(1);
% Torques_left(2)=-Torques_left(2);

Torques_des=[Torques_right;Torques_left];

end

== matlab function Control_model_10DOF_fin/Control/Inititial_Transfert/Left stance phase1/Subsystem/MATLAB Function5 ==
  data: r_vrp_W input size=3; r_DCM_W input size=3; TWR input; TWL input; lFoot parameter; dsegment parameter; new_vrp_W output; new_vrp_R output; outside output; cas output
function [new_vrp_W,new_vrp_R,outside,cas]  = support_polygon(r_vrp_W,r_DCM_W,TWR,TWL,lFoot,dsegment)

Right_foot_position=TWR(1:3,4);
Left_foot_position=TWL(1:3,4);

RWR=TWR(1:3,1:3);

R1W=Right_foot_position+RWR*[0;lFoot/2;dsegment/2];
R2W=Right_foot_position+RWR*[0;lFoot/2;-dsegment/2];
R3W=Right_foot_position+RWR*[0;-lFoot/2;-dsegment/2];
R4W=Right_foot_position+RWR*[0;-lFoot/2;dsegment/2];

L1W=Left_foot_position+RWR*[0;lFoot/2;dsegment/2];
L2W=Left_foot_position+RWR*[0;lFoot/2;-dsegment/2];
L3W=Left_foot_position+RWR*[0;-lFoot/2;-dsegment/2];
L4W=Left_foot_position+RWR*[0;-lFoot/2;dsegment/2];

% Projection on the ground
R1W(2)=0;
R2W(2)=0;
R3W(2)=0;
R4W(2)=0;

L1W(2)=0;
L2W(2)=0;
L3W(2)=0;
L4W(2)=0;

% New frame

x=1/norm(R1W-R4W)*(R1W-R4W);
y=[0;1;0];
z=1/norm(R2W-R1W)*(R2W-R1W);

R=[x,y,z];

% Points on the Right foot origin and new frame

R1=R.'*(R1W-Right_foot_position);
R2=R.'*(R2W-Right_foot_position);
R3=R.'*(R3W-Right_foot_position);
R4=R.'*(R4W-Right_foot_position);

L1=R.'*(L1W-Right_foot_position);
L2=R.'*(L2W-Right_foot_position);
L3=R.'*(L3W-Right_foot_position);
L4=R.'*(L4W-Right_foot_position);


% VRP and DCM on the left foot origin and new frame

r_vrp=R.'*(r_vrp_W-Right_foot_position);
r_DCM=R.'*(r_DCM_W-Right_foot_position);

% VRP DCM line

u=1/norm(r_DCM-r_vrp)*(r_DCM-r_vrp);

%Plane L1 L2

uL1L2=1/norm(L2-L1)*(L2-L1);
vL1L2=cross(uL1L2,y);
dL1L2=-(vL1L2(1)*L1(1)+vL1L2(2)*L1(2)+vL1L2(3)*L1(3));

tL1L2=-(vL1L2(1)*r_vrp(1)+vL1L2(2)*r_vrp(2)+vL1L2(3)*r_vrp(3)+dL1L2)/(vL1L2(1)*u(1)+vL1L2(2)*u(2)+vL1L2(3)*u(3));

%Plane L2 R2

uL2R2=1/norm(R2-L2)*(R2-L2);
vL2R2=cross(uL2R2,y);
dL2R2=-(vL2R2(1)*L2(1)+vL2R2(2)*L2(2)+vL2R2(3)*L2(3));

tL2R2=-(vL2R2(1)*r_vrp(1)+vL2R2(2)*r_vrp(2)+vL2R2(3)*r_vrp(3)+dL2R2)/(vL2R2(1)*u(1)+vL2R2(2)*u(2)+vL2R2(3)*u(3));

%Plane R2 R3

uR2R3=1/norm(R3-R2)*(R3-R2);
vR2R3=cross(uR2R3,y);
dR2R3=-(vR2R3(1)*R2(1)+vR2R3(2)*R2(2)+vR2R3(3)*R2(3));

tR2R3=-(vR2R3(1)*r_vrp(1)+vR2R3(2)*r_vrp(2)+vR2R3(3)*r_vrp(3)+dR2R3)/(vR2R3(1)*u(1)+vR2R3(2)*u(2)+vR2R3(3)*u(3));

%Plane R3 R4

uR3R4=1/norm(R4-R3)*(R4-R3);
vR3R4=cross(uR3R4,y);
dR3R4=-(vR3R4(1)*R3(1)+vR3R4(2)*R3(2)+vR3R4(3)*R3(3));

tR3R4=-(vR3R4(1)*r_vrp(1)+vR3R4(2)*r_vrp(2)+vR3R4(3)*r_vrp(3)+dR3R4)/(vR3R4(1)*u(1)+vR3R4(2)*u(2)+vR3R4(3)*u(3));

%Plane R4 L4

uR4L4=1/norm(L4-R4)*(L4-R4);
vR4L4=cross(uR4L4,y);
dR4L4=-(vR4L4(1)*R4(1)+vR4L4(2)*R4(2)+vR4L4(3)*R4(3));

tR4L4=-(vR4L4(1)*r_vrp(1)+vR4L4(2)*r_vrp(2)+vR4L4(3)*r_vrp(3)+dR4L4)/(vR4L4(1)*u(1)+vR4L4(2)*u(2)+vR4L4(3)*u(3));

%Plane L4 L1

uL4L1=1/norm(L1-L4)*(L1-L4);
vL4L1=cross(uL4L1,y);
dL4L1=-(vL4L1(1)*L4(1)+vL4L1(2)*L4(2)+vL4L1(3)*L4(3));

tL4L1=-(vL4L1(1)*r_vrp(1)+vL4L1(2)*r_vrp(2)+vL4L1(3)*r_vrp(3)+dL4L1)/(vL4L1(1)*u(1)+vL4L1(2)*u(2)+vL4L1(3)*u(3));



%Calcul affine line
a1=(L1(3)-R1(3))/(L1(1)-R1(1));
b1=R1(3)-a1*R1(1);

a2=(L2(3)-R2(3))/(L2(1)-R2(1));
b2=R2(3)-a2*R2(1);

a3=(L3(3)-R3(3))/(L3(1)-R3(1));
b3=R3(3)-a3*R3(1);

a4=(L4(3)-R4(3))/(L4(1)-R4(1));
b4=R4(3)-a4*R4(1);

a5=(r_vrp(3)-r_DCM(3))/(r_vrp(1)-r_DCM(1));
b5=r_DCM(3)-a5*r_DCM(1);

outside=1;

if r_vrp(3)>L1(3) && r_vrp(1)<L1(1) && r_vrp(3)<R3(3) && r_vrp(1)>R3(1)
    outside=0;
    if r_vrp(1)>1/a2*(r_vrp(3)-b2) || r_vrp(1)<1/a4*(r_vrp(3)+b4)
        outside=1;
    end
end



cas=0;

new_vrp=r_vrp;

if outside==1
    if r_vrp(1)<R3(1)
        cas=1;
        new_vrp=u*tR3R4+r_vrp;
        if new_vrp(3)>R3(3)
            cas=2;
            new_vrp=u*tR2R3+r_vrp;
            if new_vrp(1)>R2(1)
                cas=3;
                new_vrp(1)=R2(1);
                new_vrp(3)=R2(3);
            elseif new_vrp(1)<R3(1)
                cas=4;
                new_vrp(1)=R3(1);
                new_vrp(3)=R3(3);
            end
        elseif new_vrp(3)<R4(3)
            cas=5;
            new_vrp=u*tR4L4+r_vrp;
            if new_vrp(3)>R4(3)
                cas=6;
                new_vrp(1)=R4(1);
                new_vrp(3)=R4(3);
            elseif new_vrp(3)<L4(3)
                cas=7;
                new_vrp=u*tL4L1+r_vrp;
                if new_vrp(1)>L1(1)
                    cas=8;
                    new_vrp(1)=L1(1);
                    new_vrp(3)=L1(3);
                elseif new_vrp(1)<L4(1)
                    cas=9;
                    new_vrp(1)=L4(1);
                    new_vrp(3)=L4(3);
                end
            end
        end
    elseif r_vrp(1)>L1(1)
        cas=10;
        new_vrp=u*tL1L2+r_vrp;
        if new_vrp(3)<L1(3)
            cas=11;
            new_vrp=u*tL4L1+r_vrp;
            if new_vrp(1)<L4(1)
                cas=12;
                new_vrp(1)=L4(1);
                new_vrp(3)=L4(3);
            elseif new_vrp(1)>L1(1)
                cas=13;
                new_vrp(1)=L1(1);
                new_vrp(3)=L1(3);
            end
        elseif new_vrp(3)>L2(3)
            cas=14;
            new_vrp=u*tL2R2+r_vrp;
            if new_vrp(3)<L2(3)
                cas=15;
                new_vrp(1)=L2(1);
                new_vrp(3)=L2(3);
            elseif new_vrp(3)>R2(3)
                cas=16;
                new_vrp=u*tR2R3+r_vrp;
                if new_vrp(1)>R2(1)
                    cas=17;
                    new_vrp(1)=R2(1);
                    new_vrp(3)=R2(3);
                elseif new_vrp(1)<R3(1)
                    cas=18;
                    new_vrp(1)=R3(1);
                    new_vrp(3)=R3(3);
                end
            end
        end
    elseif r_vrp(3)>R3(3) && r_vrp(1)<L1(1) && r_vrp(1)>R3(1)
        cas=19;
        new_vrp=u*tR2R3+r_vrp;
        if new_vrp(1)<R3(1)
            cas=20;
            new_vrp(1)=R3(1);
            new_vrp(3)=R3(3);
        elseif new_vrp(1)>R2(1)
            cas=21;
            new_vrp=u*tL2R2+r_vrp;
            if new_vrp(1)<R2(1)
                cas=22;
                new_vrp(1)=R2(1);
                new_vrp(3)=R2(3);
            elseif new_vrp(1)>L2(1)
                cas=23;
                new_vrp(1)=L2(1);
                new_vrp(3)=L2(2);
            end
        end
    elseif r_vrp(3)<L1(3) && r_vrp(1)<L1(1) && r_vrp(1)>R3(1)
        cas=24;
        new_vrp=u*tL4L1+r_vrp;
        if new_vrp(1)>L1(1)
            cas=25;
            new_vrp(1)=L1(1);
            new_vrp(3)=L1(3);
        elseif new_vrp(1)<L4(1)
            cas=26;
            new_vrp=u*tR4L4+r_vrp;
            if new_vrp(1)>L4(1)
                cas=27;
                new_vrp(1)=L4(1);
                new_vrp(3)=L4(3);
            elseif new_vrp(1)<R4(1)
                cas=28;
                new_vrp(1)=R4(1);
                new_vrp(3)=R4(3);
            end
        end
    elseif r_vrp(1)<1/a4*(r_vrp(3)-b3) && r_vrp(3)>L4(3) && r_vrp(1)>R3(1)
        cas=29;
        new_vrp=u*tR4L4+r_vrp;
        if new_vrp(3)<L4(3)
            cas=30;
            new_vrp(1)=L4(1);
            new_vrp(3)=L4(3);
        elseif new_vrp(3)>R4(3)
            cas=31;
            new_vrp(1)=R4(1);
            new_vrp(3)=R4(3);
        end
    elseif r_vrp(1)>1/a2*(r_vrp(3)-b2) && r_vrp(1)<L1(1) && r_vrp(3)<R3(3)
        cas=32;
        new_vrp=u*tL2R2+r_vrp;
        if new_vrp(1)>L2(1)
            cas=33;
            new_vrp(1)=L2(1);
            new_vrp(3)=L2(3);
        elseif new_vrp(3)>R2(3)
            cas=34;
            new_vrp(1)=R2(1);
            new_vrp(3)=R2(3);
        end
    end
end


new_vrp_W=R*new_vrp+Right_foot_position;
new_vrp_R=RWR.'*(new_vrp_W-Right_foot_position);

== matlab function Control_model_10DOF_fin/Control/Inititial_Transfert/Left stance phase1/Subsystem/VRP based DCM tracking control ==
  data: r_extrapolated_CoM input double size=[3 1]; r_vrp output double size=[3 1]; DCM_velocity input double size=[3 1]; height_vrp parameter double size=1; DCM_position input double size=[3 1]; K_DCM parameter double size=[3 3]
function r_vrp = vrp_calcul(r_extrapolated_CoM,DCM_velocity,height_vrp, DCM_position, K_DCM)
%Gravity
g=9.81;
% K_DCM=2*[1 0 0;
% 0 1 0;
% 0 0 1];

r_vrp=r_extrapolated_CoM+K_DCM*sqrt(height_vrp/g)*(r_extrapolated_CoM-DCM_position)-sqrt(height_vrp/g)*DCM_velocity;

== matlab function Control_model_10DOF_fin/Control/Inititial_Transfert/Left stance phase1/Subsystem/extrapolated CoM calcul ==
  data: CoM_position input double size=[3 1]; r_extrapolate_CoM output double size=[3 1]; CoM_velocity input double size=[3 1]; height_vrp parameter double size=1
function r_extrapolate_CoM = DCM_calcul(CoM_position,CoM_velocity,height_vrp)
%Gravity
g=9.81;
r_extrapolate_CoM=CoM_position+sqrt(height_vrp/g)*CoM_velocity;

== matlab function Control_model_10DOF_fin/Control/Inititial_Transfert/Right stance phase/Subsystem/MATLAB Function ==
  data: r_vrp input double size=[3 1]; Force_des output double size=[3 1]; r_CoM input double size=[3 1]; mass parameter double size=1; height_vrp parameter double size=1
function Force_des = Force_transformation(r_vrp,r_CoM, mass, height_vrp)
g=9.81;
Force_des = mass*g/height_vrp*(r_CoM-(r_vrp-[0;height_vrp;0]));
